simulink model "class17"  (R2025b)
settings: Solver=VariableStepAuto  StartTime=0.0  StopTime=10.0  RelTol=1e-3
values from neighbouring files (symbols this model uses):
  c = 10    [Obs_temp.m]    (also in class12.m; class13.m; class14.m; class15.m)
  k = 1000    [Obs_temp.m]    (also in class12.m; class13.m; class14.m; class15.m)
  m = 1    [CtP.m]    (also in Obs_temp.m = 10; class10.m; class11.m; class12.m = 10)
settings Model: Creator=anish  LastModifiedBy=anish

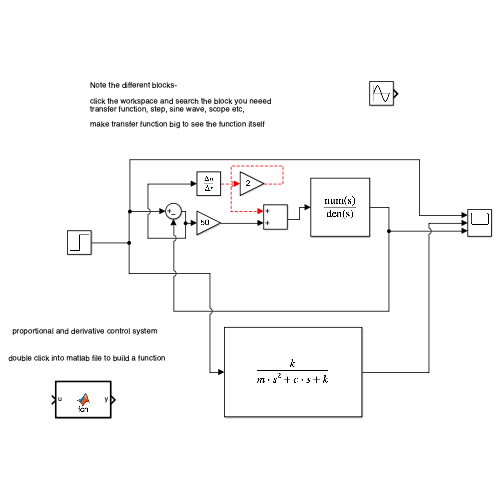
[thumbnail: Simulink's stored preview of the top-level diagram]
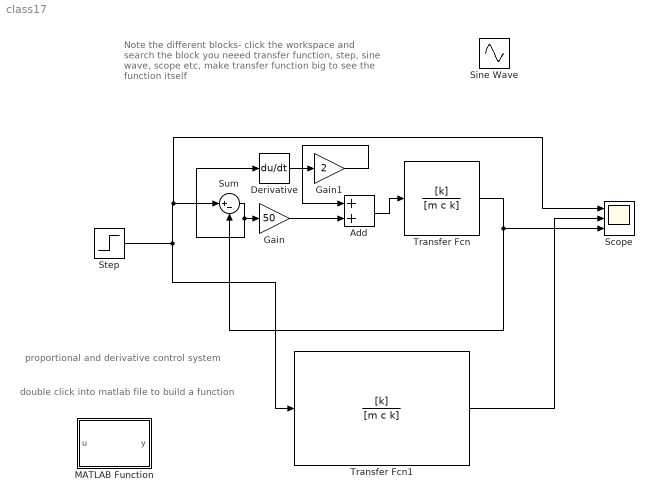
== system class17 ==
  note: double click into matlab file to build a function
  note: proportional and derivative control system
  note: Note the different blocks-
      |
      | click the workspace and search the block you neeed
      | transfer function, step, sine wave, scope etc,
      |
      | make transfer function big to see the function itself
  Add : Sum
  Derivative : Derivative
  Gain : Gain  Gain=50
  Gain1 : Gain  Gain=2
  MATLAB Function : MATLAB Function  TreatAsAtomicUnit=on
  Scope : Scope  NumInputPorts=3
      settings: SampleTime=0.01  ActiveDisplayYMinimum=-0.49402813027823522  ActiveDisplayYMaximum=1.9766697690911719
  Sine Wave : Sin  Frequency=50  SampleTime=0
  Step : Step  SampleTime=0
  Sum : Sum  Inputs=|+-
  Transfer Fcn : TransferFcn  Numerator=[k]  Denominator=[m c k]
  Transfer Fcn1 : TransferFcn  Numerator=[k]  Denominator=[m c k]
  wires:
  Transfer Fcn/1 -> Sum/2, Scope/3
  Step/1 -> Scope/1, Sum/1, Transfer Fcn1/1
  Sum/1 -> Derivative/1, Gain/1
  Transfer Fcn1/1 -> Scope/2
  Derivative/1 -> Gain1/1
  Gain1/1 -> Add/1
  Gain/1 -> Add/2
  Add/1 -> Transfer Fcn/1

== matlab function class17/MATLAB Function ==
  data: u input; y output
function y = fcn(u)

y = u;
